simulink model "MdXX_DoneChk"  (R2024b)
settings: Solver=FixedStepDiscrete  StartTime=0.0  StopTime=10.0  FixedStep=0.01  RelTol=1e-3
undefined symbols (not defined in the file or in its folder): KeSMSuVehicleModelConfig_Val
libraries: simulink x44
(part 1 of 3)
settings Model: Creator=sn2xws  LastModifiedBy=sn55gm
settings Model: ModifiedHistory=|
  | 2024.5.8 557 eze 模式及复位模式变更
  | 2024.8.23 v3.0.1 增加Lug6sDone 的信号连接
  | 2024.9.25 V3.0.2 Md2，Md3，Md29 的左右modeDone应保持至all结束
  | 2024.9.29 V3.0.3 增加Md56退出
  | 2024.10.14 V3.0.4 新增Md57 ，Md58
  | 2024.12.18 V3.8.0 CR955881 <REQ_MSM_868>
  | 25.7.8 V3.13.0 新增Md61 62
settings SolverCC: AlgebraicLoopSolver=TrustRegion
settings DataIOCC: SaveFormat=StructureWithTime  ReturnWorkspaceOutputs=off
settings OptimizationCC: DefaultParameterBehavior=Inlined  EnhancedBackFolding=on  PassReuseOutputArgsAs=Individual arguments  ZeroExternalMemoryAtStartup=off  ZeroInternalMemoryAtStartup=off  OptimizeBlockOrder=speed  DifferentSizesBufferReuse=on  OptimizationCustomize=off  EfficientTunableParamExpr=on
settings DebuggingCC: ParameterTunabilityLossMsg=error  UnconnectedInputMsg=warning  UnconnectedOutputMsg=warning  UnconnectedLineMsg=warning  ArithmeticOperatorsInVariantConditions=warning
settings ModelReferenceCC: EnableRefExpFcnMdlSchedulingChecks=on
settings SFSimCC: MATLABDynamicMemAlloc=off  CustomCodeUndefinedFunction=UseInterfaceOnly
settings RTWCC: Description=AUTOSAR  SystemTargetFile=autosar.tlc  GenCodeOnly=on  TemplateMakefile=ert_default_tmf  GenerateReport=on  IncludeHyperlinkInReport=on  LaunchReport=on  DataTypeReplacement=CDataTypesFixedWidth  GenerateTraceInfo=on  GenerateTraceReport=on  GenerateTraceReportSl=on  GenerateTraceReportSf=on  GenerateTraceReportEml=on  GenerateCodeMetricsReport=on  GPUComputeCapability=3.5
settings CodeAppCC: ForceParamTrailComments=on  IgnoreCustomStorageClasses=off  OperatorAnnotations=on  SimulinkDataObjDesc=on  SFDataObjDesc=on  InsertBlockDesc=on
settings STFCustomTargetCC: TargetLangStandard=C99 (ISO)  MultiwordLength=256  ParMdlRefBuildCompliant=on  CompOptLevelCompliant=on  IncludeMdlTerminateFcn=off  CombineOutputUpdateFcns=on  SuppressErrorStatus=on  ERTCustomFileBanners=on  SupportNonFinite=off  SupportComplex=off  SupportContinuousTime=off  SupportNonInlinedSFcns=off  RemoveResetFunc=on  MATLABClassNameForMDSCustomization=Simulink.SoftwareTarget.ERTCustomization  AutosarCompliant=on  UseToolchainInfoCompliant=on  LookupTableObjectStructAxisOrder=2,1,3,4,...  LUTObjectStructOrderEvenSpacing=Size,Table,Breakpoints  SystemTargetFile=autosar.tlc
settings ERTTargetCC: TargetLangStandard=C99 (ISO)  ConcurrentExecutionCompliant=off  IncludeMdlTerminateFcn=off  SuppressErrorStatus=on  SupportNonFinite=off  SupportComplex=off  ModelStepFunctionPrototypeControlCompliant=off  CPPClassGenCompliant=off  AutosarCompliant=on  LookupTableObjectStructAxisOrder=2,1,3,4,...  LUTObjectStructOrderEvenSpacing=Size,Table,Breakpoints  ERTCustomFileTemplate=example_file_process.tlc  ERTFilePackagingFormat=Compact  BooleanTrueId=TRUE  BooleanFalseId=FALSE  DynamicArrayContainerType=coder::array

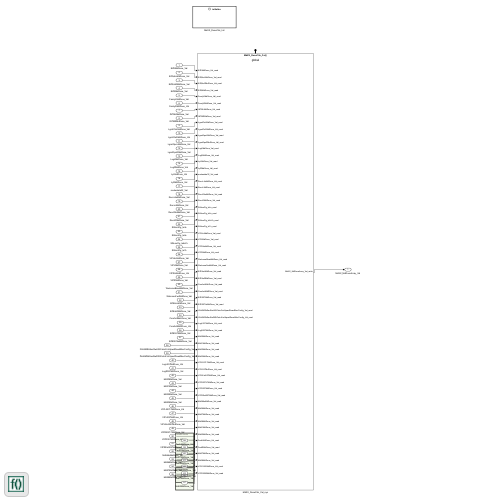
[thumbnail: Simulink's stored preview of the top-level diagram]
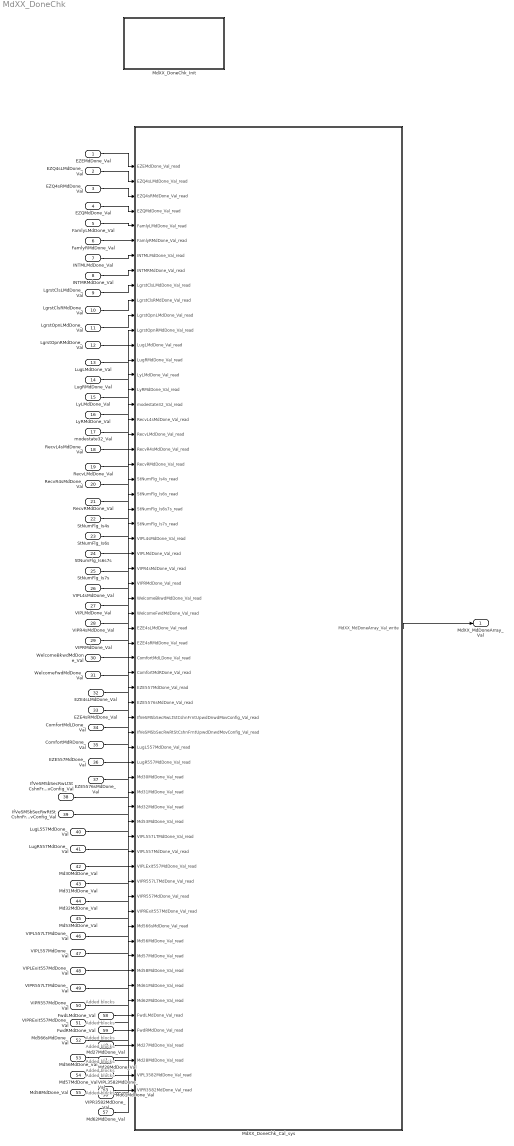
== system MdXX_DoneChk ==
  note: Added blocks
  note: Added blocks
  note: Added blocks
  note: Added blocks
  note: Added blocks
  note: Added blocks
  note: Added blocks
  note: Added blocks
  EZEMdDone_Val : Inport  OutDataTypeStr=uint8  PortDimensions=1
  EZQ4sLMdDone_Val : Inport  Port=2  OutDataTypeStr=uint8  PortDimensions=1
  EZQ4sRMdDone_Val : Inport  Port=3  OutDataTypeStr=uint8  PortDimensions=1
  EZQMdDone_Val : Inport  Port=4  OutDataTypeStr=uint8  PortDimensions=1
  FamlyLMdDone_Val : Inport  Port=5  OutDataTypeStr=uint8  PortDimensions=1
  FamlyRMdDone_Val : Inport  Port=6  OutDataTypeStr=uint8  PortDimensions=1
  INTMLMdDone_Val : Inport  Port=7  OutDataTypeStr=uint8  PortDimensions=1
  INTMRMdDone_Val : Inport  Port=8  OutDataTypeStr=uint8  PortDimensions=1
  LgrstClsLMdDone_Val : Inport  Port=9  OutDataTypeStr=uint8  PortDimensions=1
  LgrstClsRMdDone_Val : Inport  Port=10  OutDataTypeStr=uint8  PortDimensions=1
  LgrstOpnLMdDone_Val : Inport  Port=11  OutDataTypeStr=uint8  PortDimensions=1
  LgrstOpnRMdDone_Val : Inport  Port=12  OutDataTypeStr=uint8  PortDimensions=1
  LugLMdDone_Val : Inport  Port=13  OutDataTypeStr=uint8  PortDimensions=1
  LugRMdDone_Val : Inport  Port=14  OutDataTypeStr=uint8  PortDimensions=1
  LyLMdDone_Val : Inport  Port=15  OutDataTypeStr=uint8  PortDimensions=1
  LyRMdDone_Val : Inport  Port=16  OutDataTypeStr=uint8  PortDimensions=1
  modestate32_Val : Inport  Port=17  OutDataTypeStr=uint32  PortDimensions=1
  RecvL4sMdDone_Val : Inport  Port=18  OutDataTypeStr=uint8  PortDimensions=1
  RecvLMdDone_Val : Inport  Port=19  OutDataTypeStr=uint8  PortDimensions=1
  RecvR4sMdDone_Val : Inport  Port=20  OutDataTypeStr=uint8  PortDimensions=1
  RecvRMdDone_Val : Inport  Port=21  OutDataTypeStr=uint8  PortDimensions=1
  StNumFlg_Is4s : Inport  Port=22  OutDataTypeStr=boolean  PortDimensions=1
  StNumFlg_Is6s : Inport  Port=23  OutDataTypeStr=boolean  PortDimensions=1
  StNumFlg_Is6s7s : Inport  Port=24  OutDataTypeStr=boolean  PortDimensions=1
  StNumFlg_Is7s : Inport  Port=25  OutDataTypeStr=boolean  PortDimensions=1
  VIPL4sMdDone_Val : Inport  Port=26  OutDataTypeStr=uint8  PortDimensions=1
  VIPLMdDone_Val : Inport  Port=27  OutDataTypeStr=uint8  PortDimensions=1
  VIPR4sMdDone_Val : Inport  Port=28  OutDataTypeStr=uint8  PortDimensions=1
  VIPRMdDone_Val : Inport  Port=29  OutDataTypeStr=uint8  PortDimensions=1
  WelcomeBkwdMdDone_Val : Inport  Port=30  OutDataTypeStr=uint8  PortDimensions=1
  WelcomeFwdMdDone_Val : Inport  Port=31  OutDataTypeStr=uint8  PortDimensions=1
  EZE4sLMdDone_Val : Inport  Port=32  OutDataTypeStr=uint8  PortDimensions=1
  EZE4sRMdDone_Val : Inport  Port=33  OutDataTypeStr=uint8  PortDimensions=1
  ComfortMdLDone_Val : Inport  Port=34  OutDataTypeStr=uint8  PortDimensions=1
  ComfortMdRDone_Val : Inport  Port=35  OutDataTypeStr=uint8  PortDimensions=1
  EZE557MdDone_Val : Inport  Port=36  OutDataTypeStr=uint8  PortDimensions=1
  EZE5576sMdDone_Val : Inport  Port=37  OutDataTypeStr=uint8  PortDimensions=1
  IfVeSMSbSecRwLtStCshnFrntUpwdDnwdMovConfig_Val : Inport  Port=38  OutDataTypeStr=boolean  PortDimensions=1
  IfVeSMSbSecRwRtStCshnFrntUpwdDnwdMovConfig_Val : Inport  Port=39  OutDataTypeStr=boolean  PortDimensions=1
  LugL557MdDone_Val : Inport  Port=40  OutDataTypeStr=uint8  PortDimensions=1
  LugR557MdDone_Val : Inport  Port=41  OutDataTypeStr=uint8  PortDimensions=1
  Md30MdDone_Val : Inport  Port=42  OutDataTypeStr=uint8  PortDimensions=1
  Md31MdDone_Val : Inport  Port=43  OutDataTypeStr=uint8  PortDimensions=1
  Md32MdDone_Val : Inport  Port=44  OutDataTypeStr=uint8  PortDimensions=1
  Md53MdDone_Val : Inport  Port=45  OutDataTypeStr=uint8  PortDimensions=1
  VIPL557LTMdDone_Val : Inport  Port=46  OutDataTypeStr=uint8  PortDimensions=1
  VIPL557MdDone_Val : Inport  Port=47  OutDataTypeStr=uint8  PortDimensions=1
  VIPLExit557MdDone_Val : Inport  Port=48  OutDataTypeStr=uint8  PortDimensions=1
  VIPR557LTMdDone_Val : Inport  Port=49  OutDataTypeStr=uint8  PortDimensions=1
  VIPR557MdDone_Val : Inport  Port=50  OutDataTypeStr=uint8  PortDimensions=1
  VIPRExit557MdDone_Val : Inport  Port=51  OutDataTypeStr=uint8  PortDimensions=1
  Md566sMdDone_Val : Inport  Port=52  OutDataTypeStr=uint8  PortDimensions=1
  Md56MdDone_Val : Inport  Port=53  OutDataTypeStr=uint8  PortDimensions=1
  Md57MdDone_Val : Inport  Port=54  OutDataTypeStr=uint8  PortDimensions=1
  Md58MdDone_Val : Inport  Port=55  OutDataTypeStr=uint8  PortDimensions=1
  Md61MdDone_Val : Inport  Port=56  OutDataTypeStr=uint8  PortDimensions=1
  Md62MdDone_Val : Inport  Port=57  OutDataTypeStr=uint8  PortDimensions=1
  FwdLMdDone_Val : Inport  Port=58  OutDataTypeStr=uint8  PortDimensions=1
  FwdRMdDone_Val : Inport  Port=59  OutDataTypeStr=uint8  PortDimensions=1
  Md27MdDone_Val : Inport  Port=60  OutDataTypeStr=uint8  PortDimensions=1
  Md28MdDone_Val : Inport  Port=61  OutDataTypeStr=uint8  PortDimensions=1
  VIPL3582MdDone_Val : Inport  Port=62  OutDataTypeStr=uint8  PortDimensions=1
  VIPR3582MdDone_Val : Inport  Port=63  OutDataTypeStr=uint8  PortDimensions=1
  MdXX_DoneChk_Cal_sys : Subsystem
  MdXX_DoneChk_Init : Subsystem
  MdXX_MdDoneArray_Val : Outport  OutDataTypeStr=uint8  PortDimensions=32  VectorParamsAs1DForOutWhenUnconnected=off
  wires:
  EZEMdDone_Val/1 -> MdXX_DoneChk_Cal_sys/1(EZEMdDone_Val_read)
  EZQ4sLMdDone_Val/1 -> MdXX_DoneChk_Cal_sys/2(EZQ4sLMdDone_Val_read)
  EZQ4sRMdDone_Val/1 -> MdXX_DoneChk_Cal_sys/3(EZQ4sRMdDone_Val_read)
  EZQMdDone_Val/1 -> MdXX_DoneChk_Cal_sys/4(EZQMdDone_Val_read)
  FamlyLMdDone_Val/1 -> MdXX_DoneChk_Cal_sys/5(FamlyLMdDone_Val_read)
  FamlyRMdDone_Val/1 -> MdXX_DoneChk_Cal_sys/6(FamlyRMdDone_Val_read)
  INTMLMdDone_Val/1 -> MdXX_DoneChk_Cal_sys/7(INTMLMdDone_Val_read)
  INTMRMdDone_Val/1 -> MdXX_DoneChk_Cal_sys/8(INTMRMdDone_Val_read)
  LgrstClsLMdDone_Val/1 -> MdXX_DoneChk_Cal_sys/9(LgrstClsLMdDone_Val_read)
  LgrstClsRMdDone_Val/1 -> MdXX_DoneChk_Cal_sys/10(LgrstClsRMdDone_Val_read)
  LgrstOpnLMdDone_Val/1 -> MdXX_DoneChk_Cal_sys/11(LgrstOpnLMdDone_Val_read)
  LgrstOpnRMdDone_Val/1 -> MdXX_DoneChk_Cal_sys/12(LgrstOpnRMdDone_Val_read)
  LugLMdDone_Val/1 -> MdXX_DoneChk_Cal_sys/13(LugLMdDone_Val_read)
  LugRMdDone_Val/1 -> MdXX_DoneChk_Cal_sys/14(LugRMdDone_Val_read)
  LyLMdDone_Val/1 -> MdXX_DoneChk_Cal_sys/15(LyLMdDone_Val_read)
  LyRMdDone_Val/1 -> MdXX_DoneChk_Cal_sys/16(LyRMdDone_Val_read)
  modestate32_Val/1 -> MdXX_DoneChk_Cal_sys/17(modestate32_Val_read)
  RecvL4sMdDone_Val/1 -> MdXX_DoneChk_Cal_sys/18(RecvL4sMdDone_Val_read)
  RecvLMdDone_Val/1 -> MdXX_DoneChk_Cal_sys/19(RecvLMdDone_Val_read)
  RecvR4sMdDone_Val/1 -> MdXX_DoneChk_Cal_sys/20(RecvR4sMdDone_Val_read)
  RecvRMdDone_Val/1 -> MdXX_DoneChk_Cal_sys/21(RecvRMdDone_Val_read)
  StNumFlg_Is4s/1 -> MdXX_DoneChk_Cal_sys/22(StNumFlg_Is4s_read)
  StNumFlg_Is6s/1 -> MdXX_DoneChk_Cal_sys/23(StNumFlg_Is6s_read)
  StNumFlg_Is6s7s/1 -> MdXX_DoneChk_Cal_sys/24(StNumFlg_Is6s7s_read)
  StNumFlg_Is7s/1 -> MdXX_DoneChk_Cal_sys/25(StNumFlg_Is7s_read)
  VIPL4sMdDone_Val/1 -> MdXX_DoneChk_Cal_sys/26(VIPL4sMdDone_Val_read)
  VIPLMdDone_Val/1 -> MdXX_DoneChk_Cal_sys/27(VIPLMdDone_Val_read)
  VIPR4sMdDone_Val/1 -> MdXX_DoneChk_Cal_sys/28(VIPR4sMdDone_Val_read)
  VIPRMdDone_Val/1 -> MdXX_DoneChk_Cal_sys/29(VIPRMdDone_Val_read)
  WelcomeBkwdMdDone_Val/1 -> MdXX_DoneChk_Cal_sys/30(WelcomeBkwdMdDone_Val_read)
  WelcomeFwdMdDone_Val/1 -> MdXX_DoneChk_Cal_sys/31(WelcomeFwdMdDone_Val_read)
  MdXX_DoneChk_Cal_sys/1(MdXX_MdDoneArray_Val_write) -> MdXX_MdDoneArray_Val/1
  EZE4sLMdDone_Val/1 -> MdXX_DoneChk_Cal_sys/32(EZE4sLMdDone_Val_read)
  EZE4sRMdDone_Val/1 -> MdXX_DoneChk_Cal_sys/33(EZE4sRMdDone_Val_read)
  ComfortMdLDone_Val/1 -> MdXX_DoneChk_Cal_sys/34(ComfortMdLDone_Val_read)
  ComfortMdRDone_Val/1 -> MdXX_DoneChk_Cal_sys/35(ComfortMdRDone_Val_read)
  EZE557MdDone_Val/1 -> MdXX_DoneChk_Cal_sys/36(EZE557MdDone_Val_read)
  EZE5576sMdDone_Val/1 -> MdXX_DoneChk_Cal_sys/37(EZE5576sMdDone_Val_read)
  IfVeSMSbSecRwLtStCshnFrntUpwdDnwdMovConfig_Val/1 -> MdXX_DoneChk_Cal_sys/38(IfVeSMSbSecRwLtStCshnFrntUpwdDnwdMovConfig_Val_read)
  IfVeSMSbSecRwRtStCshnFrntUpwdDnwdMovConfig_Val/1 -> MdXX_DoneChk_Cal_sys/39(IfVeSMSbSecRwRtStCshnFrntUpwdDnwdMovConfig_Val_read)
  LugL557MdDone_Val/1 -> MdXX_DoneChk_Cal_sys/40(LugL557MdDone_Val_read)
  LugR557MdDone_Val/1 -> MdXX_DoneChk_Cal_sys/41(LugR557MdDone_Val_read)
  Md30MdDone_Val/1 -> MdXX_DoneChk_Cal_sys/42(Md30MdDone_Val_read)
  Md31MdDone_Val/1 -> MdXX_DoneChk_Cal_sys/43(Md31MdDone_Val_read)
  Md32MdDone_Val/1 -> MdXX_DoneChk_Cal_sys/44(Md32MdDone_Val_read)
  Md53MdDone_Val/1 -> MdXX_DoneChk_Cal_sys/45(Md53MdDone_Val_read)
  VIPL557LTMdDone_Val/1 -> MdXX_DoneChk_Cal_sys/46(VIPL557LTMdDone_Val_read)
  VIPL557MdDone_Val/1 -> MdXX_DoneChk_Cal_sys/47(VIPL557MdDone_Val_read)
  VIPLExit557MdDone_Val/1 -> MdXX_DoneChk_Cal_sys/48(VIPLExit557MdDone_Val_read)
  VIPR557LTMdDone_Val/1 -> MdXX_DoneChk_Cal_sys/49(VIPR557LTMdDone_Val_read)
  VIPR557MdDone_Val/1 -> MdXX_DoneChk_Cal_sys/50(VIPR557MdDone_Val_read)
  VIPRExit557MdDone_Val/1 -> MdXX_DoneChk_Cal_sys/51(VIPRExit557MdDone_Val_read)
  Md566sMdDone_Val/1 -> MdXX_DoneChk_Cal_sys/52(Md566sMdDone_Val_read)
  Md56MdDone_Val/1 -> MdXX_DoneChk_Cal_sys/53(Md56MdDone_Val_read)
  Md57MdDone_Val/1 -> MdXX_DoneChk_Cal_sys/54(Md57MdDone_Val_read)
  Md58MdDone_Val/1 -> MdXX_DoneChk_Cal_sys/55(Md58MdDone_Val_read)
  Md61MdDone_Val/1 -> MdXX_DoneChk_Cal_sys/56(Md61MdDone_Val_read)
  Md62MdDone_Val/1 -> MdXX_DoneChk_Cal_sys/57(Md62MdDone_Val_read)
  FwdLMdDone_Val/1 -> MdXX_DoneChk_Cal_sys/58(FwdLMdDone_Val_read)
  FwdRMdDone_Val/1 -> MdXX_DoneChk_Cal_sys/59(FwdRMdDone_Val_read)
  Md27MdDone_Val/1 -> MdXX_DoneChk_Cal_sys/60(Md27MdDone_Val_read)
  Md28MdDone_Val/1 -> MdXX_DoneChk_Cal_sys/61(Md28MdDone_Val_read)
  VIPL3582MdDone_Val/1 -> MdXX_DoneChk_Cal_sys/62(VIPL3582MdDone_Val_read)
  VIPR3582MdDone_Val/1 -> MdXX_DoneChk_Cal_sys/63(VIPR3582MdDone_Val_read)

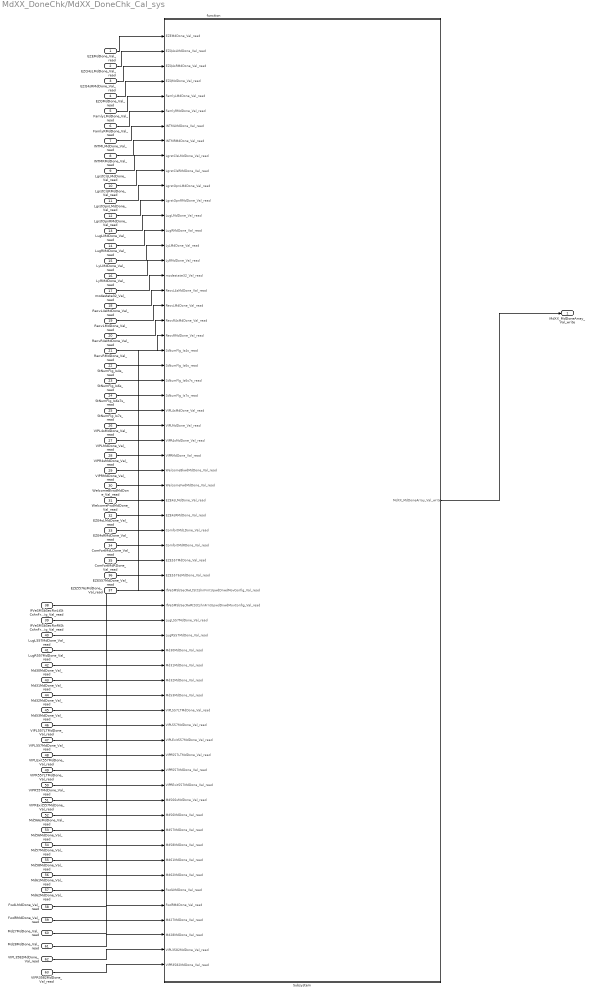
== system MdXX_DoneChk/MdXX_DoneChk_Cal_sys ==
  EZEMdDone_Val_read : Inport
  EZQ4sLMdDone_Val_read : Inport  Port=2
  EZQ4sRMdDone_Val_read : Inport  Port=3
  EZQMdDone_Val_read : Inport  Port=4
  FamlyLMdDone_Val_read : Inport  Port=5
  FamlyRMdDone_Val_read : Inport  Port=6
  INTMLMdDone_Val_read : Inport  Port=7
  INTMRMdDone_Val_read : Inport  Port=8
  LgrstClsLMdDone_Val_read : Inport  Port=9
  LgrstClsRMdDone_Val_read : Inport  Port=10
  LgrstOpnLMdDone_Val_read : Inport  Port=11
  LgrstOpnRMdDone_Val_read : Inport  Port=12
  LugLMdDone_Val_read : Inport  Port=13
  LugRMdDone_Val_read : Inport  Port=14
  LyLMdDone_Val_read : Inport  Port=15
  LyRMdDone_Val_read : Inport  Port=16
  modestate32_Val_read : Inport  Port=17
  RecvL4sMdDone_Val_read : Inport  Port=18
  RecvLMdDone_Val_read : Inport  Port=19
  RecvR4sMdDone_Val_read : Inport  Port=20
  RecvRMdDone_Val_read : Inport  Port=21
  StNumFlg_Is4s_read : Inport  Port=22
  StNumFlg_Is6s_read : Inport  Port=23
  StNumFlg_Is6s7s_read : Inport  Port=24
  StNumFlg_Is7s_read : Inport  Port=25
  VIPL4sMdDone_Val_read : Inport  Port=26
  VIPLMdDone_Val_read : Inport  Port=27
  VIPR4sMdDone_Val_read : Inport  Port=28
  VIPRMdDone_Val_read : Inport  Port=29
  WelcomeBkwdMdDone_Val_read : Inport  Port=30
  WelcomeFwdMdDone_Val_read : Inport  Port=31
  EZE4sLMdDone_Val_read : Inport  Port=32
  EZE4sRMdDone_Val_read : Inport  Port=33
  ComfortMdLDone_Val_read : Inport  Port=34
  ComfortMdRDone_Val_read : Inport  Port=35
  EZE557MdDone_Val_read : Inport  Port=36
  EZE5576sMdDone_Val_read : Inport  Port=37
  IfVeSMSbSecRwLtStCshnFrntUpwdDnwdMovConfig_Val_read : Inport  Port=38
  IfVeSMSbSecRwRtStCshnFrntUpwdDnwdMovConfig_Val_read : Inport  Port=39
  LugL557MdDone_Val_read : Inport  Port=40
  LugR557MdDone_Val_read : Inport  Port=41
  Md30MdDone_Val_read : Inport  Port=42
  Md31MdDone_Val_read : Inport  Port=43
  Md32MdDone_Val_read : Inport  Port=44
  Md53MdDone_Val_read : Inport  Port=45
  VIPL557LTMdDone_Val_read : Inport  Port=46
  VIPL557MdDone_Val_read : Inport  Port=47
  VIPLExit557MdDone_Val_read : Inport  Port=48
  VIPR557LTMdDone_Val_read : Inport  Port=49
  VIPR557MdDone_Val_read : Inport  Port=50
  VIPRExit557MdDone_Val_read : Inport  Port=51
  Md566sMdDone_Val_read : Inport  Port=52
  Md56MdDone_Val_read : Inport  Port=53
  Md57MdDone_Val_read : Inport  Port=54
  Md58MdDone_Val_read : Inport  Port=55
  Md61MdDone_Val_read : Inport  Port=56
  Md62MdDone_Val_read : Inport  Port=57
  FwdLMdDone_Val_read : Inport  Port=58
  FwdRMdDone_Val_read : Inport  Port=59
  Md27MdDone_Val_read : Inport  Port=60
  Md28MdDone_Val_read : Inport  Port=61
  VIPL3582MdDone_Val_read : Inport  Port=62
  VIPR3582MdDone_Val_read : Inport  Port=63
  function : TriggerPort  TriggerType=function-call  IsSimulinkFunction=on  FunctionName=MdXX_DoneChk_Cal  VariantControl=(inherit)
  Subsystem : Subsystem
  MdXX_MdDoneArray_Val_write : Outport  VectorParamsAs1DForOutWhenUnconnected=off
      settings: EnsureOutportIsVirtual=on
  wires:
  EZEMdDone_Val_read/1 -> Subsystem/1(EZEMdDone_Val_read)
  EZQ4sLMdDone_Val_read/1 -> Subsystem/2(EZQ4sLMdDone_Val_read)
  EZQ4sRMdDone_Val_read/1 -> Subsystem/3(EZQ4sRMdDone_Val_read)
  EZQMdDone_Val_read/1 -> Subsystem/4(EZQMdDone_Val_read)
  FamlyLMdDone_Val_read/1 -> Subsystem/5(FamlyLMdDone_Val_read)
  FamlyRMdDone_Val_read/1 -> Subsystem/6(FamlyRMdDone_Val_read)
  INTMLMdDone_Val_read/1 -> Subsystem/7(INTMLMdDone_Val_read)
  INTMRMdDone_Val_read/1 -> Subsystem/8(INTMRMdDone_Val_read)
  LgrstClsLMdDone_Val_read/1 -> Subsystem/9(LgrstClsLMdDone_Val_read)
  LgrstClsRMdDone_Val_read/1 -> Subsystem/10(LgrstClsRMdDone_Val_read)
  LgrstOpnLMdDone_Val_read/1 -> Subsystem/11(LgrstOpnLMdDone_Val_read)
  LgrstOpnRMdDone_Val_read/1 -> Subsystem/12(LgrstOpnRMdDone_Val_read)
  LugLMdDone_Val_read/1 -> Subsystem/13(LugLMdDone_Val_read)
  LugRMdDone_Val_read/1 -> Subsystem/14(LugRMdDone_Val_read)
  LyLMdDone_Val_read/1 -> Subsystem/15(LyLMdDone_Val_read)
  LyRMdDone_Val_read/1 -> Subsystem/16(LyRMdDone_Val_read)
  modestate32_Val_read/1 -> Subsystem/17(modestate32_Val_read)
  RecvL4sMdDone_Val_read/1 -> Subsystem/18(RecvL4sMdDone_Val_read)
  RecvLMdDone_Val_read/1 -> Subsystem/19(RecvLMdDone_Val_read)
  RecvR4sMdDone_Val_read/1 -> Subsystem/20(RecvR4sMdDone_Val_read)
  RecvRMdDone_Val_read/1 -> Subsystem/21(RecvRMdDone_Val_read)
  StNumFlg_Is4s_read/1 -> Subsystem/22(StNumFlg_Is4s_read)
  StNumFlg_Is6s_read/1 -> Subsystem/23(StNumFlg_Is6s_read)
  StNumFlg_Is6s7s_read/1 -> Subsystem/24(StNumFlg_Is6s7s_read)
  StNumFlg_Is7s_read/1 -> Subsystem/25(StNumFlg_Is7s_read)
  VIPL4sMdDone_Val_read/1 -> Subsystem/26(VIPL4sMdDone_Val_read)
  VIPLMdDone_Val_read/1 -> Subsystem/27(VIPLMdDone_Val_read)
  VIPR4sMdDone_Val_read/1 -> Subsystem/28(VIPR4sMdDone_Val_read)
  VIPRMdDone_Val_read/1 -> Subsystem/29(VIPRMdDone_Val_read)
  WelcomeBkwdMdDone_Val_read/1 -> Subsystem/30(WelcomeBkwdMdDone_Val_read)
  WelcomeFwdMdDone_Val_read/1 -> Subsystem/31(WelcomeFwdMdDone_Val_read)
  Subsystem/1(MdXX_MdDoneArray_Val_write) -> MdXX_MdDoneArray_Val_write/1
  EZE4sLMdDone_Val_read/1 -> Subsystem/32(EZE4sLMdDone_Val_read)
  EZE4sRMdDone_Val_read/1 -> Subsystem/33(EZE4sRMdDone_Val_read)
  ComfortMdLDone_Val_read/1 -> Subsystem/34(ComfortMdLDone_Val_read)
  ComfortMdRDone_Val_read/1 -> Subsystem/35(ComfortMdRDone_Val_read)
  EZE557MdDone_Val_read/1 -> Subsystem/36(EZE557MdDone_Val_read)
  EZE5576sMdDone_Val_read/1 -> Subsystem/37(EZE5576sMdDone_Val_read)
  IfVeSMSbSecRwLtStCshnFrntUpwdDnwdMovConfig_Val_read/1 -> Subsystem/38(IfVeSMSbSecRwLtStCshnFrntUpwdDnwdMovConfig_Val_read)
  IfVeSMSbSecRwRtStCshnFrntUpwdDnwdMovConfig_Val_read/1 -> Subsystem/39(IfVeSMSbSecRwRtStCshnFrntUpwdDnwdMovConfig_Val_read)
  LugL557MdDone_Val_read/1 -> Subsystem/40(LugL557MdDone_Val_read)
  LugR557MdDone_Val_read/1 -> Subsystem/41(LugR557MdDone_Val_read)
  Md30MdDone_Val_read/1 -> Subsystem/42(Md30MdDone_Val_read)
  Md31MdDone_Val_read/1 -> Subsystem/43(Md31MdDone_Val_read)
  Md32MdDone_Val_read/1 -> Subsystem/44(Md32MdDone_Val_read)
  Md53MdDone_Val_read/1 -> Subsystem/45(Md53MdDone_Val_read)
  VIPL557LTMdDone_Val_read/1 -> Subsystem/46(VIPL557LTMdDone_Val_read)
  VIPL557MdDone_Val_read/1 -> Subsystem/47(VIPL557MdDone_Val_read)
  VIPLExit557MdDone_Val_read/1 -> Subsystem/48(VIPLExit557MdDone_Val_read)
  VIPR557LTMdDone_Val_read/1 -> Subsystem/49(VIPR557LTMdDone_Val_read)
  VIPR557MdDone_Val_read/1 -> Subsystem/50(VIPR557MdDone_Val_read)
  VIPRExit557MdDone_Val_read/1 -> Subsystem/51(VIPRExit557MdDone_Val_read)
  Md566sMdDone_Val_read/1 -> Subsystem/52(Md566sMdDone_Val_read)
  Md56MdDone_Val_read/1 -> Subsystem/53(Md56MdDone_Val_read)
  Md57MdDone_Val_read/1 -> Subsystem/54(Md57MdDone_Val_read)
  Md58MdDone_Val_read/1 -> Subsystem/55(Md58MdDone_Val_read)
  Md61MdDone_Val_read/1 -> Subsystem/56(Md61MdDone_Val_read)
  Md62MdDone_Val_read/1 -> Subsystem/57(Md62MdDone_Val_read)
  FwdLMdDone_Val_read/1 -> Subsystem/58(FwdLMdDone_Val_read)
  FwdRMdDone_Val_read/1 -> Subsystem/59(FwdRMdDone_Val_read)
  Md27MdDone_Val_read/1 -> Subsystem/60(Md27MdDone_Val_read)
  Md28MdDone_Val_read/1 -> Subsystem/61(Md28MdDone_Val_read)
  VIPL3582MdDone_Val_read/1 -> Subsystem/62(VIPL3582MdDone_Val_read)
  VIPR3582MdDone_Val_read/1 -> Subsystem/63(VIPR3582MdDone_Val_read)

== system MdXX_DoneChk/MdXX_DoneChk_Init ==
  note: Added blocks
  Event Listener : EventListener  EventName=reset
  PA_KeSMSuVehicleModelConfig_Val : Constant  Value=KeSMSuVehicleModelConfig_Val
  Terminator_1 : Terminator
  wires:
  PA_KeSMSuVehicleModelConfig_Val/1 -> Terminator_1/1
